simulink model "main"  (R2022b)
settings: Solver=FixedStepDiscrete  StartTime=0.0  StopTime=50  FixedStep=0.005  RelTol=1e-3
settings Model: ExtModeTrigDuration=2  Creator=F64236C  LastModifiedBy=F64236C
settings OptimizationCC: EnhancedBackFolding=on  PassReuseOutputArgsAs=Individual arguments  ZeroExternalMemoryAtStartup=off  ZeroInternalMemoryAtStartup=off  MaxStackSize=64  OptimizeBlockOrder=speed  DifferentSizesBufferReuse=on  OptimizationCustomize=off  EfficientTunableParamExpr=on
settings DebuggingCC: ParameterTunabilityLossMsg=error
settings HardwareCC: ProdBitPerPointer=32  ProdBitPerSizeT=32  ProdBitPerPtrDiffT=32  ProdLargestAtomicInteger=Long  ProdLargestAtomicFloat=Double  ProdWordSize=32  ProdHWDeviceType=ARM Compatible->ARM Cortex
settings SFSimCC: MATLABDynamicMemAlloc=off
settings RTWCC: Description=Embedded Coder  SystemTargetFile=ert.tlc  HardwareBoard=ESP32-WROOM(Arduino Compatible)  TLCOptions="-aInlineSetEventsForThisBaseRateFcn=TLC_FALSE -aSuppressMultiTaskScheduler=TLC_FALSE  -aRateBasedStepFcn=0"  TemplateMakefile=ert_default_tmf  Toolchain=ESP32  BuildConfiguration=Faster Runs
settings CodeAppCC: ForceParamTrailComments=on  IgnoreCustomStorageClasses=off  OperatorAnnotations=on  SimulinkDataObjDesc=on  SFDataObjDesc=on  InsertBlockDesc=on
settings ERTTargetCC: SupportContinuousTime=on  SupportVariableSizeSignals=on  ExtModeTransport=3  ExtModeStaticAlloc=on  ExtModeAutomaticAllocSize=off  ExtModeStaticAllocSize=65536  ExtModeMexFile=ext_xcp  ExtModeIntrfLevel=Level2 - Open

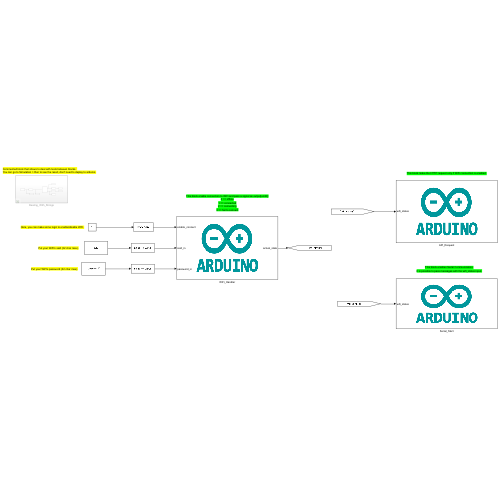
[thumbnail: Simulink's stored preview of the top-level diagram]
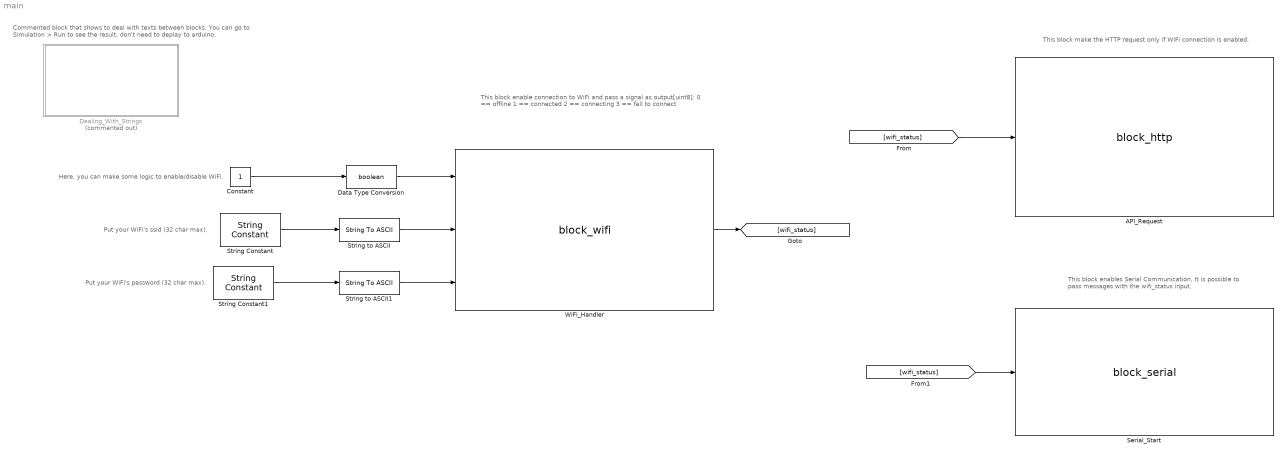
== system main ==
  note: Commented block that shows to deal with texts between blocks.
      | You can go to Simulation > Run to see the result, don't need to deplay to arduino.
  note: This block enable connection to WiFi and pass a signal as output[uint8]:
      | 0 == offline
      | 1 == connected
      | 2 == connecting
      | 3 == fail to connect
  note: Here, you can make some logic to enable/disable WiFi.
  note: Put your WiFi's ssid (32 char max).
  note: Put your WiFi's password (32 char max).
  note: This block enables Serial Communication.
      | It is possible to pass messages with the wifi_status input.
  note: This block make the HTTP request only if WiFi connection is enabled.
  API_Request : S-Function  FunctionName=block_http  SFunctionModules=block_http_wrapper.cpp  SFunctionDeploymentMode=off  EnableBusSupport=off  mask(S-Function Builder){}
      mask help: Simulink:masks:SFunctionBuilder_MD
      mask init:
      | val = [[.9  0.75 0.75 1 1 .9 .9 1]',[1 1 0.75 0.75 .9 .9 1 .9]'];try , sys = get_param(gcb,'SfunBuilderFcnName');if isempty(sys), sys = get_param(gcb,'FunctionName'); end,catch, sys = get_param(gcb,'FunctionName'); end
      settings: CopyFcn=set_param(gcbh,'LinkStatus','none')  OpenFcn=sfunctionwizard(gcbh)
      mask Display:
      | image('../imgs/arduino_logo.png');
      | port_label('input',1,'wifi_status')
  Constant : Constant
  Data Type Conversion : DataTypeConversion  OutDataTypeStr=boolean  SaturateOnIntegerOverflow=off  RndMeth=Floor
  Dealing_With_Strings : Subsystem  Commented=on
  Serial_Start : S-Function  FunctionName=block_serial  SFunctionModules=block_serial_wrapper.cpp  SFunctionDeploymentMode=off  EnableBusSupport=off  mask(S-Function Builder){}
      mask help: Simulink:masks:SFunctionBuilder_MD
      mask init: same as main/API_Request
      settings: CopyFcn=set_param(gcbh,'LinkStatus','none')  OpenFcn=sfunctionwizard(gcbh)
      mask Display:
      | image('../imgs/arduino_logo.png');
      | port_label('input',1,'wifi_status')
  String Constant : StringConstant  String="\"ssid\""
  String Constant1 : StringConstant  String="\"password\""
  String to ASCII : StringToASCII  OutputVectorSize=32
  String to ASCII1 : StringToASCII  OutputVectorSize=32
  WiFi_Handler : S-Function  FunctionName=block_wifi  SFunctionModules=block_wifi_wrapper.cpp  SFunctionDeploymentMode=off  EnableBusSupport=off  mask(S-Function Builder){}
      mask help: Simulink:masks:SFunctionBuilder_MD
      mask init: same as main/API_Request
      settings: CopyFcn=set_param(gcbh,'LinkStatus','none')  OpenFcn=sfunctionwizard(gcbh)
      mask Display:
      | image('../imgs/arduino_logo.png');
      | 
      | port_label('input',1,'enable_connect')
      | port_label('input',2,'ssid_in')
      | port_label('input',3,'password_in')
      | port_label('output',1,'actual_state')
  wires:
  Data Type Conversion/1 -> WiFi_Handler/1
  Constant/1 -> Data Type Conversion/1
  String Constant/1 -> String to ASCII/1
  String to ASCII/1 -> WiFi_Handler/2
  String Constant1/1 -> String to ASCII1/1
  String to ASCII1/1 -> WiFi_Handler/3
  WiFi_Handler/1 -> [wifi_status]
  [wifi_status] -> API_Request/1
  [wifi_status] -> Serial_Start/1

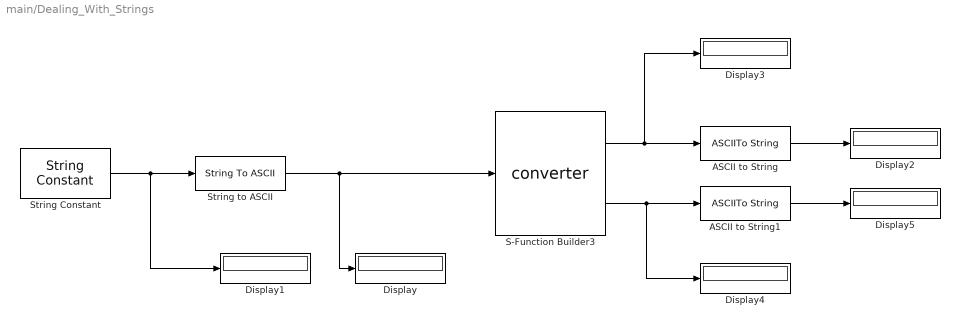
== system main/Dealing_With_Strings ==
  ASCII to String : ASCIIToString
  ASCII to String1 : ASCIIToString
  Display{,1..5} (6 alike) : Display
  S-Function Builder3 : S-Function  FunctionName=converter  SFunctionModules=converter_wrapper.cpp  SFunctionDeploymentMode=off  EnableBusSupport=off  mask(S-Function Builder){}
      mask help: Simulink:masks:SFunctionBuilder_MD
      mask init: same as main/API_Request
      settings: CopyFcn=set_param(gcbh,'LinkStatus','none')  OpenFcn=sfunctionwizard(gcbh)
      mask Display:
      | plot(val(:,1),val(:,2))
      | disp(sys)
      | port_label('input',1,'in')
      | port_label('output',1,'out')
      | port_label('output',2,'saida_t')
  String Constant : StringConstant
  String to ASCII : StringToASCII  OutputVectorSize=32
  wires:
  ASCII to String1/1 -> Display5/1
  String Constant/1 -> String to ASCII/1, Display1/1
  String to ASCII/1 -> Display/1, S-Function Builder3/1
  S-Function Builder3/1 -> Display3/1, ASCII to String/1
  S-Function Builder3/2 -> Display4/1, ASCII to String1/1
  ASCII to String/1 -> Display2/1
